simulink model "integralsimmm"  (R2023a)
settings: Solver=VariableStepAuto  StartTime=0.0  StopTime=10.0  RelTol=1e-3
values from neighbouring files (symbols this model uses):
  k = 1/(R*C)    (= 59.8211348069)    [ode_RC.m]
settings Model: Creator=jackr  LastModifiedBy=jackr

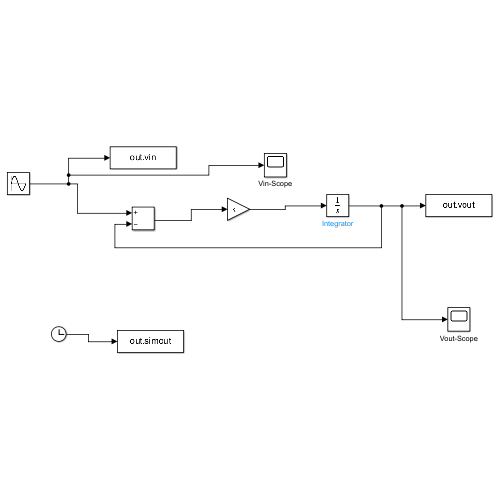
[thumbnail: Simulink's stored preview of the top-level diagram]
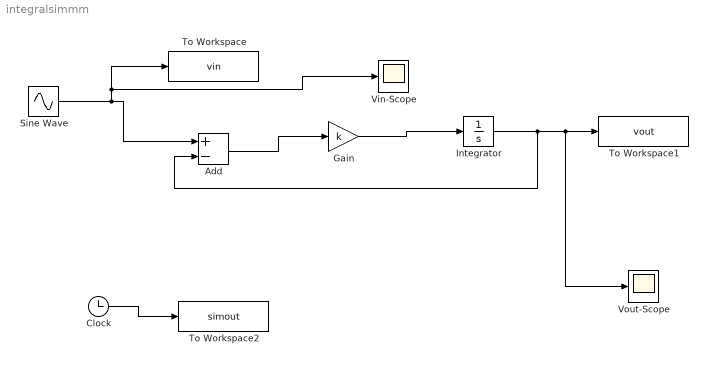
== system integralsimmm ==
  Add : Sum  Inputs=+-
  Clock : Clock
  Gain : Gain  Gain=k
  Integrator : Integrator
  Sine Wave : Sin  Frequency=2*pi * 50  Phase=pi/2  SampleTime=0
  To Workspace : ToWorkspace  VariableName=vin  SaveFormat=Timeseries  SampleTime=-1
  To Workspace1 : ToWorkspace  VariableName=vout  SaveFormat=Timeseries  SampleTime=-1
  To Workspace2 : ToWorkspace  VariableName=simout  SaveFormat=Timeseries  SampleTime=-1
  Vin-Scope : Scope
  Vout-Scope : Scope
  wires:
  Add/1 -> Gain/1
  Gain/1 -> Integrator/1
  Integrator/1 -> Add/2, Vout-Scope/1, To Workspace1/1
  Clock/1 -> To Workspace2/1
  Sine Wave/1 -> Vin-Scope/1, To Workspace/1, Add/1
